simulink model "evaluate_estim_model_stability"  (R2023b)
settings: Solver=VariableStepAuto  StartTime=0.0  StopTime=24  MaxStep=0.01  MinStep=0.001  RelTol=1e-3
values from neighbouring files (symbols this model uses):
  A = [0 0 1; -par(1)*par(2) 0 -par(2)*par(3); 0 0 0]    [myfunc.m]
  B = [0; par(2); 0]    [myfunc.m]
  C = [1 0 0]    [myfunc.m]
undefined symbols (not defined in the file or in its folder): E
settings Model: Creator=hdt  LastModifiedBy=hdt
settings SolverCC: AutoInsertRateTranBlk=on

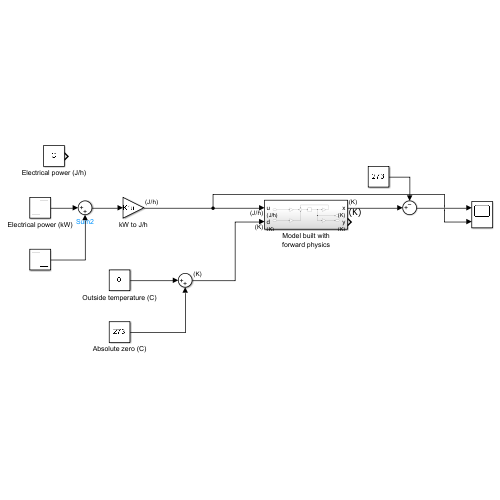
[thumbnail: Simulink's stored preview of the top-level diagram]
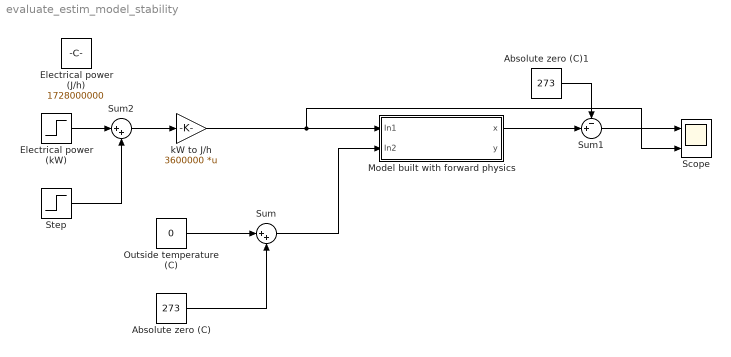
== system evaluate_estim_model_stability ==
  Absolute zero (C) : Constant  Value=273
  Absolute zero (C)1 : Constant  Value=273
  Electrical power (J/h) : Constant  Value=1728000000
  Electrical power (kW) : Step  Time=5  After=48  SampleTime=0
  Model built with forward physics : Subsystem
  Outside temperature (C) : Constant  Value=0
  Scope : Scope  NumInputPorts=2
  Step : Step  Time=5.05  After=-48  SampleTime=0
  Sum : Sum  Inputs=|++
  Sum1 : Sum  Inputs=-+|
  Sum2 : Sum  Inputs=|++
  kW to J/h : Gain  Gain=3600000  Multiplication=Matrix(K*u)
  wires:
  Electrical power (kW)/1 -> Sum2/1
  Absolute zero (C)/1 -> Sum/2
  Outside temperature (C)/1 -> Sum/1
  Sum/1 -> Model built with forward physics/2(In2)
  Model built with forward physics/1(x) -> Sum1/2
  Absolute zero (C)1/1 -> Sum1/1
  Sum1/1 -> Scope/1
  kW to J/h/1 -> Scope/2, Model built with forward physics/1(In1)
  Sum2/1 -> kW to J/h/1
  Step/1 -> Sum2/2

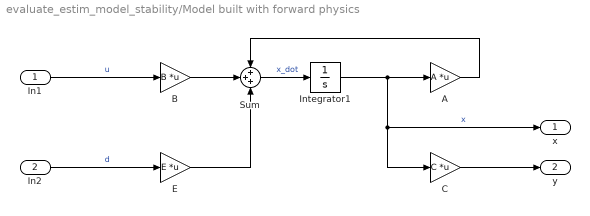
== system evaluate_estim_model_stability/Model built with forward physics ==
  In1 : Inport  Unit=J/h
  In2 : Inport  Port=2  Unit=K
  A : Gain  Gain=A  Multiplication=Matrix(K*u)
  B : Gain  Gain=B  Multiplication=Matrix(K*u)
  C : Gain  Gain=C  Multiplication=Matrix(K*u)
  E : Gain  Gain=E  Multiplication=Matrix(K*u)
  Integrator1 : Integrator  InitialCondition=[293;297]
  Sum : Sum  Inputs=+++
  x : Outport  Unit=K
  y : Outport  Port=2  Unit=K
  wires:
  In1/1 -> B/1  "u"
  B/1 -> Sum/2
  A/1 -> Sum/1
  Sum/1 -> Integrator1/1  "x_dot"
  Integrator1/1 -> A/1, C/1, x/1  "x"
  E/1 -> Sum/3
  In2/1 -> E/1  "d"
  C/1 -> y/1
